simulink model "linmodel_eq2"  (R2019a)
settings: Solver=VariableStepAuto  StartTime=0.0  StopTime=30  RelTol=1e-3
InitFcn:
  | lin_discr_model
undefined symbols (not defined in the file): A_eq2, B, C, Continuous, T, Time
libraries: ctrlSharedLib x1
settings Model: Creator=jessi  LastModifiedBy=jessi

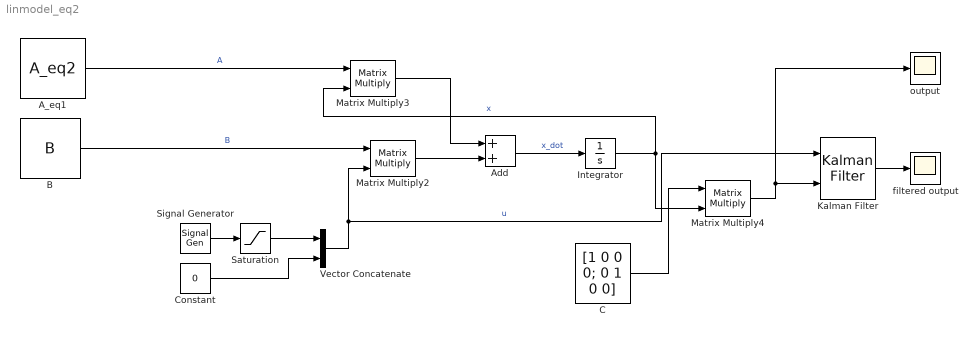
== system linmodel_eq2 ==
  A_eq1 : Constant  Value=A_eq2
  Add : Sum
  B : Constant  Value=B
  C : Constant  Value=|
      | [1 0 0 0;
      | 0 1 0 0]
  Constant : Constant  Value=0
  Integrator : Integrator  InitialCondition=[0;0;0;0]
  Kalman Filter : ctrlSharedLib/Kalman Filter  TimeDomain=Continuous-Time  UseCurrentEstimator=on  ModelSource=Individual A, B, C, D matrices  ModelSourceVariable=ss(0.95,1,1,0,1)  A=A_eq2  B=B  C=C  D=0  NumberOfStates=1  NumberOfInputs=1  NumberOfOutputs=1  InitialEstimateSource=Dialog  X0=[0;0;0;0]  P0=10  UseK=off  UseGH=off  NumberOfProcessNoiseInputs=1  G=1  TimeInvariantG=on  H=0  TimeInvariantH=on  Q=diag([0,0,0,0])  TimeInvariantQ=on  R=diag([0.1, 0.1])  TimeInvariantR=on  N=0  TimeInvariantN=on  AddInputPort=on  AddEnablePort=off  OutputEstimatedY=off  OutputP=off  Ts=T
      settings: SourceProductBaseCode=CT
  Matrix Multiply2 : Product  Multiplication=Matrix(*)
  Matrix Multiply3 : Product  Multiplication=Matrix(*)
  Matrix Multiply4 : Product  Multiplication=Matrix(*)
  Saturation : Saturate  UpperLimit=1  LowerLimit=-1
  Signal Generator : SignalGenerator  WaveForm=square  Amplitude=0.3
  Vector Concatenate : Concatenate
  filtered output : Scope
  output : Scope
  wires:
  B/1 -> Matrix Multiply2/1  "B"
  Matrix Multiply2/1 -> Add/2
  A_eq1/1 -> Matrix Multiply3/1  "A"
  Add/1 -> Integrator/1  "x_dot"
  Integrator/1 -> Matrix Multiply3/2, Matrix Multiply4/2  "x"
  Matrix Multiply3/1 -> Add/1
  Matrix Multiply4/1 -> Kalman Filter/2, output/1
  Signal Generator/1 -> Saturation/1
  Constant/1 -> Vector Concatenate/2
  Vector Concatenate/1 -> Kalman Filter/1, Matrix Multiply2/2  "u"
  C/1 -> Matrix Multiply4/1
  Saturation/1 -> Vector Concatenate/1
  Kalman Filter/1 -> filtered output/1
